simulink model "PDgrav"  (R2018b)
settings: Solver=FixedStepAuto  StartTime=0.0  StopTime=tfin  FixedStep=timeStep  MaxStep=1e-4  RelTol=1e-3
values from neighbouring files (symbols this model uses):
  kd = wn*damp*2    (= 28.5)    [es_1_circle.m]    (also in es_1_line.m = 57; initIDctrl.m = 32)
  kp = wn^2    (= 225)    [es_1_circle.m]    (also in es_1_line.m = 900; initIDctrl.m = 400)
  qq = ikine6s(p560,TTc)    [es_1_circle.m]    (also in es_1_line.m = ikine6s(p560,TTl))
  tfin = 5    [es_1_circle.m]    (also in es_1_line.m = 2; initIDctrl.m = 2; initSMctrl.m = 2)
libraries: roblocks x2
settings Model: Creator=Brus  LastModifiedBy=Brus

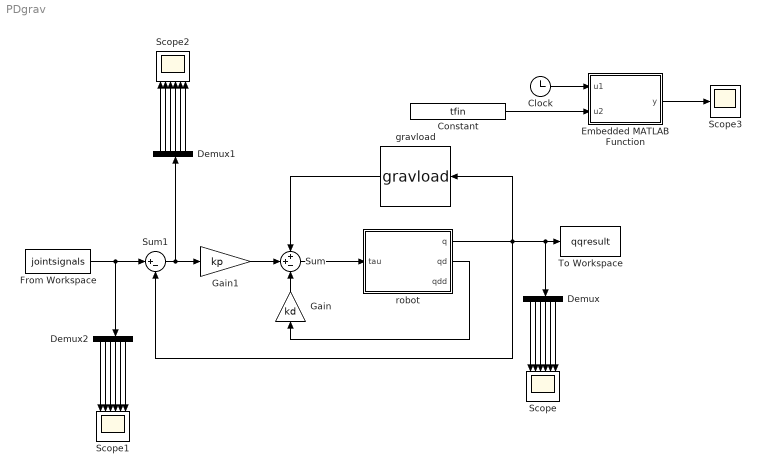
== system PDgrav ==
  Clock : Clock
  Constant : Constant  Value=tfin
  Demux : Demux  Outputs=6
  Demux1 : Demux  Outputs=6
  Demux2 : Demux  Outputs=6
  Embedded MATLAB Function : MATLAB Function  TreatAsAtomicUnit=on
  From Workspace : FromWorkspace  VariableName=jointsignals  SampleTime=0
  Gain : Gain  Gain=kd
  Gain1 : Gain  Gain=kp
  Scope : Scope  NumInputPorts=6
  Scope1 : Scope  NumInputPorts=6
  Scope2 : Scope  NumInputPorts=6
  Scope3 : Scope
  Sum : Sum  Inputs=++-
  Sum1 : Sum  Inputs=|+-
  To Workspace : ToWorkspace  VariableName=qqresult  SaveFormat=Timeseries  SampleTime=-1
  gravload : roblocks/Arm/gravload  robot=p560
  robot : Subsystem
  wires:
  Gain/1 -> Sum/3
  Gain1/1 -> Sum/2
  Demux/6 -> Scope/6
  Demux/5 -> Scope/5
  Demux/4 -> Scope/4
  Demux/2 -> Scope/2
  Demux/3 -> Scope/3
  Demux/1 -> Scope/1
  Demux2/5 -> Scope1/5
  Demux2/6 -> Scope1/6
  Demux2/4 -> Scope1/4
  Demux2/1 -> Scope1/1
  Demux2/3 -> Scope1/3
  Demux2/2 -> Scope1/2
  Demux1/5 -> Scope2/5
  Demux1/6 -> Scope2/6
  Demux1/4 -> Scope2/4
  Demux1/1 -> Scope2/1
  Demux1/3 -> Scope2/3
  Demux1/2 -> Scope2/2
  From Workspace/1 -> Demux2/1, Sum1/1
  gravload/1 -> Sum/1
  Sum1/1 -> Demux1/1, Gain1/1
  robot/1(q) -> To Workspace/1, Demux/1, gravload/1, Sum1/2
  Sum/1 -> robot/1(tau)
  robot/2(qd) -> Gain/1
  Constant/1 -> Embedded MATLAB Function/2(u2)
  Clock/1 -> Embedded MATLAB Function/1(u1)
  Embedded MATLAB Function/1(y) -> Scope3/1

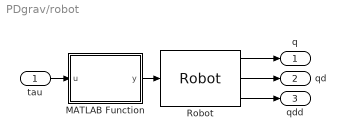
== system PDgrav/robot ==
  tau : Inport
  MATLAB Function : MATLAB Function  TreatAsAtomicUnit=on
  Robot : roblocks/Arm/Robot  robot=p560  q0=qq(1,:)
  q : Outport
  qd : Outport  Port=2
  qdd : Outport  Port=3
  wires:
  MATLAB Function/1(y) -> Robot/1
  Robot/2 -> qd/1
  Robot/1 -> q/1
  Robot/3 -> qdd/1
  tau/1 -> MATLAB Function/1(u)

== matlab function PDgrav/robot/MATLAB Function ==
  data: u input; y output
function y = checkNaN(u)
if(isnan(u))
    y=zeros(size(u));
else
    y=u;
end

== matlab function PDgrav/Embedded MATLAB Function ==
  settings: fimath=|
      | fimath(...
      | 'RoundMode', 'floor',...
      | 'OverflowMode', 'wrap',...
      | 'ProductMode', 'KeepLSB', 'ProductWordLength', 32,...
      | 'SumMode', 'KeepLSB', 'SumWordLength', 32,...
      | 'CastBeforeSum', false)
  data: u1 input; y output; u2 input
function y = fcn(u1, u2)
% This block supports an embeddable subset of the MATLAB language.
% See the help menu for details. 
coder.extrinsic('waitbar')
waitbar(u1/u2)
y = 1;
